simulink model "LQR_sistema_ecuaciones"  (R2023a)
settings: Solver=VariableStepAuto  StartTime=0.0  StopTime=500  FixedStep=0.25  RelTol=1e-3
undefined symbols (not defined in the file): A, A_model, A_motor, B, B_mag, B_model, B_motor, C_model, C_motor, D_model, D_motor, I, J, K, K1, K2, K3, Ke, Kt, La, n_cal, R_mgt, Ra, T_ext, T_max, T_max_mgt, x0
libraries: matrix_library x17, slpidlib x15, simulink_extras x6, aerolibutil x2, vrlib x2
(part 3 of 3)

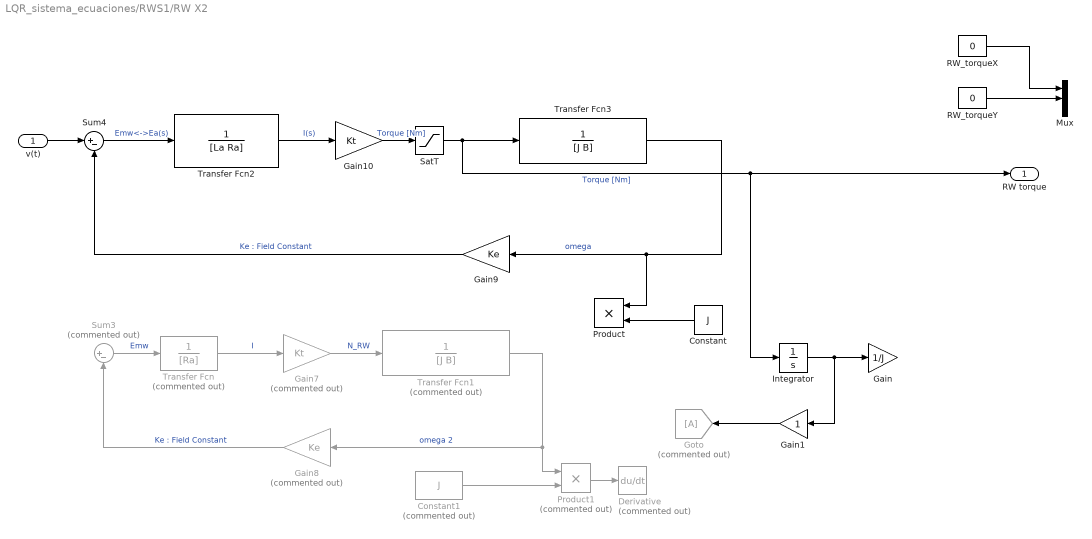
== system LQR_sistema_ecuaciones/RWS1/RW X2 ==
  v(t) : Inport
  Constant : Constant  Value=J
  Constant1 : Constant  Commented=on  Value=J
  Derivative : Derivative  Commented=on
  Gain : Gain  Gain=1/J
  Gain1 : Gain
  Gain10 : Gain  Gain=Kt
  Gain7 : Gain  Commented=on  Gain=Kt
  Gain8 : Gain  Commented=on  Gain=Ke
  Gain9 : Gain  Gain=Ke
  Goto : Goto  Commented=on
  Integrator : Integrator
  Mux : Mux  Inputs=3
  Product : Product
  Product1 : Product  Commented=on
  RW_torqueX : Constant  Value=0
  RW_torqueY : Constant  Value=0
  SatT : Saturate  UpperLimit=T_max  LowerLimit=-T_max
  Sum3 : Sum  Commented=on  Inputs=|+-
  Sum4 : Sum  Inputs=|+-
  Transfer Fcn : TransferFcn  Commented=on  Denominator=[Ra]
  Transfer Fcn1 : TransferFcn  Commented=on  Denominator=[J B]
  Transfer Fcn2 : TransferFcn  Denominator=[La Ra]
  Transfer Fcn3 : TransferFcn  Denominator=[J B]
  RW torque : Outport  VectorParamsAs1DForOutWhenUnconnected=off
  wires:
  SatT/1 -> Transfer Fcn3/1, Integrator/1, RW torque/1  "Torque [Nm]"
  Gain1/1 -> Goto/1
  Gain10/1 -> SatT/1  "Torque [Nm]"
  RW_torqueY/1 -> Mux/2
  RW_torqueX/1 -> Mux/1
  Gain8/1 -> Sum3/2  "Ke : Field Constant"
  Transfer Fcn/1 -> Gain7/1  "I"
  Sum3/1 -> Transfer Fcn/1  "Emw"
  Gain7/1 -> Transfer Fcn1/1  "N_RW"
  Transfer Fcn1/1 -> Gain8/1, Product1/1  "omega 2"
  Constant1/1 -> Product1/2
  Product1/1 -> Derivative/1
  v(t)/1 -> Sum4/1
  Integrator/1 -> Gain/1, Gain1/1
  Constant/1 -> Product/2
  Transfer Fcn3/1 -> Product/1, Gain9/1  "omega"
  Gain9/1 -> Sum4/2  "Ke : Field Constant"
  Sum4/1 -> Transfer Fcn2/1  "Emw<->Ea(s)"
  Transfer Fcn2/1 -> Gain10/1  "I(s)"

== system LQR_sistema_ecuaciones/Subsystem6/Mgt X ==
  B : Inport
  PWR : Inport  Port=2
  Cross Product : matrix_library/Cross Product
  Mgt_ejeX : Gain  Gain=[1 0 0]
  "Momento Dipolar " : Gain  Gain=n_cal*A/R_mgt
  Mgt XYZ : Outport
  wires:
  "Momento Dipolar "/1 -> Mgt_ejeX/1
  Mgt_ejeX/1 -> Cross Product/1
  Cross Product/1 -> Mgt XYZ/1  "MgtX"
  PWR/1 -> "Momento Dipolar "/1
  B/1 -> Cross Product/2

== system LQR_sistema_ecuaciones/Subsystem6/Mgt Y ==
  PWR : Inport
  B : Inport  Port=2
  Cross Product : matrix_library/Cross Product
  Mgt_ejeY : Gain  Gain=[0 1 0]
  "Momento Dipolar " : Gain  Gain=n_cal*A/R_mgt
  Mgt XYZ : Outport
  wires:
  B/1 -> Cross Product/2
  PWR/1 -> "Momento Dipolar "/1
  Cross Product/1 -> Mgt XYZ/1  "MgtX"
  Mgt_ejeY/1 -> Cross Product/1
  "Momento Dipolar "/1 -> Mgt_ejeY/1

== matlab function LQR_sistema_ecuaciones/Subsystem4/MATLAB Function ==
  data: NEDMagnetic input; RPY_Magnetic output; RPY input
function RPY_Magnetic = RPY_Magnetic(NEDMagnetic,RPY)

R = RPY(1);
P= RPY(2);
Y = RPY(3);



C_NED2ENU = [0 1 0;
             1 0 0
             0 0 -1];
C_RPY2ENU = [sin(Y)*cos(P) cos(R)*cos(Y)+sin(R)*sin(Y)*sin(P) -sin(R)*cos(Y)+cos(R)*sin(Y)*sin(P);
    cos(Y)*cos(P) -cos(R)*sin(Y)+sin(R)*cos(Y)*sin(P) sin(R)*sin(Y)+cos(R)*cos(Y)*sin(P);
    sin(P) -sin(R)*cos(P) -cos(R)*cos(P)];

C_ENU2RPY = C_RPY2ENU^-1; 

RPY_Magnetic = C_ENU2RPY*C_NED2ENU*NEDMagnetic; 


end

== matlab function LQR_sistema_ecuaciones/Subsystem2/Corrección X ==
  data: H_error input; B input; H_error output
function H_error = fcn(H_error,B)

if (B(2)> 0)
    HGain =1;
else
    HGain =- 1;

end
H_error = H_error*HGain; 
end

== matlab function LQR_sistema_ecuaciones/MATLAB Function1 ==
  settings: updateMethod=DISCRETE
  data: torques input; VoltagesXYZ output; B input; K input
function VoltagesXYZ = calVoltages(torques,B,K)

rng default % For reproducibility

Bx = B(1);
By = B(2);
Bz = B(3);

Tx = torques(1);
Ty = torques(2);
Tz = torques(3);

 F =  @(x)[0*x(1)+K*Bz*x(2)-K*By*x(3)-Tx;
          -K*Bz*x(1)+0*x(2)+K*Bx*x(3)-Ty;
          K*By*x(1)-K*Bx*x(2)+0*x(3)-Tz];

%%

VoltageFS = 7;
N = 100; % Try 10 random start points
pts = 5*rand(N,3); % Initial points are rows in pts
soln = zeros(N,3); % Allocate solution
opts = optimoptions('fsolve','Display','off','FunctionTolerance',1e-30,'Algorithm','levenberg-marquardt');
for k = 1:N
    soln(k,:) = fsolve(F,pts(k,:),opts); % Find solutions
end

idx = soln(:,1) >= -VoltageFS & soln(:,2) >= -VoltageFS & soln(:,3)>= -VoltageFS &...
    soln(:,1) <= VoltageFS & soln(:,2) <= VoltageFS & soln(:,3)<= VoltageFS;

soln_filter = soln(idx,:);
if (isempty(soln_filter))
    VoltagesXYZ = [0 0 0];

else
    VoltagesXYZ = soln_filter(1,:);
end

end

== matlab function LQR_sistema_ecuaciones/Subsystem5/MATLAB Function ==
  data: B input; magTorqueMatrix output; voltageX input; voltageY input; voltageZ input; momentoDipolar output
function [magTorqueMatrix,momentoDipolar] = magTorqueFunction(B,voltageX,voltageY,voltageZ)

%d = 1.45e-2; % Diametro mgt [m]
d = 1.45e-2; % Diametro mgt [m]
A =d^2*pi/4;

%n=sqrt(L*l/(mu_0*mu_r*A)); % # Vueltas 
n = 5412;

%R = 50.7 ;% Resistencia mgt [Ohm];
R = 30 ;% Resistencia mgt [Ohm];
ix = voltageX/R;
iy = voltageY/R;
iz = voltageZ/R;

% M = [n*ix*A n*iy*A n*iz*A]';
% 
% magTorqueMatrix = -skew(B)*M;

magTorqueMatrix_X = cross(n*ix*A*[1 0 0],B);
magTorqueMatrix_Y = cross(n*iy*A*[0 1 0],B);
magTorqueMatrix_Z = cross(n*iz*A*[0 0 1],B);
 momentoDipolar = [n*ix*A n*iy*A n*iz*A];

magTorqueMatrix = magTorqueMatrix_X+magTorqueMatrix_Y+magTorqueMatrix_Z;

== matlab function LQR_sistema_ecuaciones/MATLAB Function2 ==
  data: torques input; VoltagesXYZ output; B input; K input; tz_error output
function [VoltagesXYZ,tz_error] = calVoltages(torques,B,K)
Bx = B(1);
By = B(2);
Bz = B(3);

Tx = torques(1);
Ty = torques(2);
Tz = torques(3);

Vx = -Ty/(K*Bz);
Vy = Tx/(K*Bz);
tz_exp = -(By/Bz)*Ty-(Bx/Bz)*Tx;
tz_error = Tz - tz_exp;
VoltagesXYZ = [Vx Vy 0];
end

== matlab function LQR_sistema_ecuaciones/Subsystem/MATLAB Function ==
  data: B input; magTorqueMatrix output; voltageX input; voltageY input; voltageZ input; momentoDipolar output
function [magTorqueMatrix,momentoDipolar] = magTorqueFunction(B,voltageX,voltageY,voltageZ)

%d = 1.45e-2; % Diametro mgt [m]
d = 1.45e-2; % Diametro mgt [m]
A =d^2*pi/4;

%n=sqrt(L*l/(mu_0*mu_r*A)); % # Vueltas 
n = 5412;

%R = 50.7 ;% Resistencia mgt [Ohm];
R = 30 ;% Resistencia mgt [Ohm];
ix = voltageX/R;
iy = voltageY/R;
iz = voltageZ/R;

% M = [n*ix*A n*iy*A n*iz*A]';
% 
% magTorqueMatrix = -skew(B)*M;

magTorqueMatrix_X = cross(n*ix*A*[1 0 0],B);
magTorqueMatrix_Y = cross(n*iy*A*[0 1 0],B);
magTorqueMatrix_Z = cross(n*iz*A*[0 0 1],B);
 momentoDipolar = [n*ix*A n*iy*A n*iz*A];

magTorqueMatrix = magTorqueMatrix_X+magTorqueMatrix_Y+magTorqueMatrix_Z;

== matlab function LQR_sistema_ecuaciones/Subsystem/Corrección X ==
  data: H_error input; B input; H_error output
function H_error = fcn(H_error,B)

if (B(2)> 0)
    HGain =1;
else
    HGain =- 1;

end
H_error = H_error*HGain; 
end

== matlab function LQR_sistema_ecuaciones/Subsystem2/Corrección Y ==
  data: H_error input; B input; H_error output
function H_error = fcn(H_error,B)

if (B(1)> 0)
    HGain =-1;
else
    HGain =1 ;

end
H_error = H_error*HGain; 
end

== matlab function LQR_sistema_ecuaciones/Subsystem/Corrección Y ==
  data: H_error input; B input; H_error output
function H_error = fcn(H_error,B)

if (B(1)> 0)
    HGain =-1;
else
    HGain =1 ;

end
H_error = H_error*HGain; 
end

== matlab function LQR_sistema_ecuaciones/Subsystem1/MATLAB Function ==
  data: B input; magTorqueMatrix output; voltageX input; voltageY input; voltageZ input; momentoDipolar output
function [magTorqueMatrix,momentoDipolar] = magTorqueFunction(B,voltageX,voltageY,voltageZ)

%d = 1.45e-2; % Diametro mgt [m]
d = 1.45e-2; % Diametro mgt [m]
A =d^2*pi/4;

%n=sqrt(L*l/(mu_0*mu_r*A)); % # Vueltas 
n = 5412;

%R = 50.7 ;% Resistencia mgt [Ohm];
R = 30 ;% Resistencia mgt [Ohm];
ix = voltageX/R;
iy = voltageY/R;
iz = voltageZ/R;

% M = [n*ix*A n*iy*A n*iz*A]';
% 
% magTorqueMatrix = -skew(B)*M;

magTorqueMatrix_X = cross(n*ix*A*[1 0 0],B);
magTorqueMatrix_Y = cross(n*iy*A*[0 1 0],B);
magTorqueMatrix_Z = cross(n*iz*A*[0 0 1],B);
 momentoDipolar = [n*ix*A n*iy*A n*iz*A];

magTorqueMatrix = magTorqueMatrix_X+magTorqueMatrix_Y+magTorqueMatrix_Z;

== matlab function LQR_sistema_ecuaciones/Subsystem2/MATLAB Function ==
  data: B input; magTorqueMatrix output; voltageX input; voltageY input; voltageZ input; momentoDipolar output
function [magTorqueMatrix,momentoDipolar] = magTorqueFunction(B,voltageX,voltageY,voltageZ)

%d = 1.45e-2; % Diametro mgt [m]
d = 1.45e-2; % Diametro mgt [m]
A =d^2*pi/4;

%n=sqrt(L*l/(mu_0*mu_r*A)); % # Vueltas 
n = 5412;

%R = 50.7 ;% Resistencia mgt [Ohm];
R = 30 ;% Resistencia mgt [Ohm];
ix = voltageX/R;
iy = voltageY/R;
iz = voltageZ/R;

% M = [n*ix*A n*iy*A n*iz*A]';
% 
% magTorqueMatrix = -skew(B)*M;

magTorqueMatrix_X = cross(n*ix*A*[1 0 0],B);
magTorqueMatrix_Y = cross(n*iy*A*[0 1 0],B);
magTorqueMatrix_Z = cross(n*iz*A*[0 0 1],B);
 momentoDipolar = [n*ix*A n*iy*A n*iz*A];

magTorqueMatrix = magTorqueMatrix_X+magTorqueMatrix_Y+magTorqueMatrix_Z;

== matlab function LQR_sistema_ecuaciones/Subsystem3/MATLAB Function ==
  data: B input; magTorqueMatrix output; voltageX input; voltageY input; voltageZ input; momentoDipolar output
function [magTorqueMatrix,momentoDipolar] = magTorqueFunction(B,voltageX,voltageY,voltageZ)

%d = 1.45e-2; % Diametro mgt [m]
d = 1.45e-2; % Diametro mgt [m]
A =d^2*pi/4;

%n=sqrt(L*l/(mu_0*mu_r*A)); % # Vueltas 
n = 5412;

%R = 50.7 ;% Resistencia mgt [Ohm];
R = 30 ;% Resistencia mgt [Ohm];
ix = voltageX/R;
iy = voltageY/R;
iz = voltageZ/R;

% M = [n*ix*A n*iy*A n*iz*A]';
% 
% magTorqueMatrix = -skew(B)*M;

magTorqueMatrix_X = cross(n*ix*A*[1 0 0],B);
magTorqueMatrix_Y = cross(n*iy*A*[0 1 0],B);
magTorqueMatrix_Z = cross(n*iz*A*[0 0 1],B);
 momentoDipolar = [n*ix*A n*iy*A n*iz*A];

magTorqueMatrix = magTorqueMatrix_X+magTorqueMatrix_Y+magTorqueMatrix_Z;

== matlab function LQR_sistema_ecuaciones/Subsystem4/Extract B ==
  data: B_cal input; XYZ_Magnetic output size=[3,1]; time input
function XYZ_Magnetic = fcn(B_cal,time)

index= 1+round(time);
s = size(B_cal);
if index> s(2)
    XYZ_Magnetic = B_cal(:,s(2));
else
    XYZ_Magnetic = B_cal(:,index);
end

== matlab function LQR_sistema_ecuaciones/MATLAB Function ==
  data: torques input; VoltagesXYZ output; B input; K input
function VoltagesXYZ = calVoltages(torques,B,K)
Bx = B(1);
By = B(2);
Bz = B(3);

% Tx = torques(1);
% Ty = torques(2);
% Tz = torques(3);

A = [0 K*Bz -K*By;
    -K*Bz 0 K*Bx;
    K*By -K*Bx 0];
B = torques;


VoltagesXYZ = linsolve(A,B);
end
